simulink model "W01_S1"  (R2024b)
settings: Solver=ode4  StartTime=0  StopTime=T_final  FixedStep=h  RelTol=1e-3
undefined symbols (not defined in the file or in its folder): beta_c, mp, n0, rp, V_c, x0
settings Model: Creator=admin  LastModifiedBy=admin
settings DataIOCC: ReturnWorkspaceOutputs=off

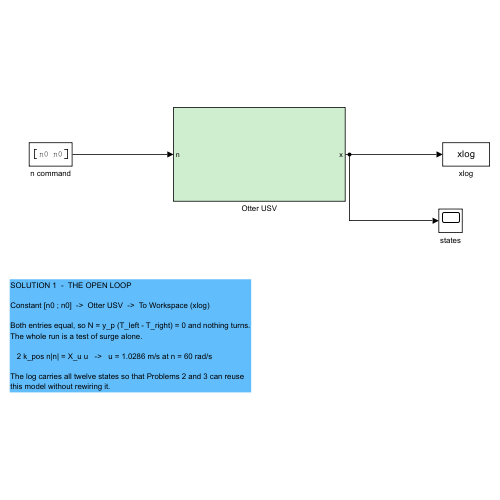
[thumbnail: Simulink's stored preview of the top-level diagram]
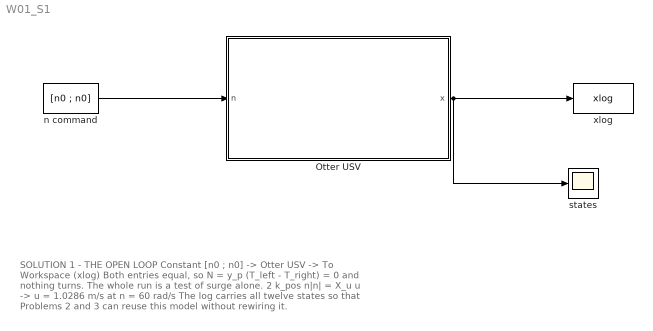
== system W01_S1 ==
  note: SOLUTION 1  -  THE OPEN LOOP
      |
      | Constant [n0 ; n0]  ->  Otter USV  ->  To Workspace (xlog)
      |
      | Both entries equal, so N = y_p (T_left - T_right) = 0 and nothing turns.
      | The whole run is a test of surge alone.
      |
      |    2 k_pos n|n| = X_u u   ->   u = 1.0286 m/s at n = 60 rad/s
      |
      | The log carries all twelve states so that Problems 2 and 3 can reuse
      | this model without rewiring it.
  Otter USV : Subsystem
  n command : Constant  Value=[n0 ; n0]
  states : Scope
  xlog : ToWorkspace  VariableName=xlog  SaveFormat=Structure With Time  SampleTime=-1
  wires:
  n command/1 -> Otter USV/1(n)
  Otter USV/1(x) -> xlog/1, states/1

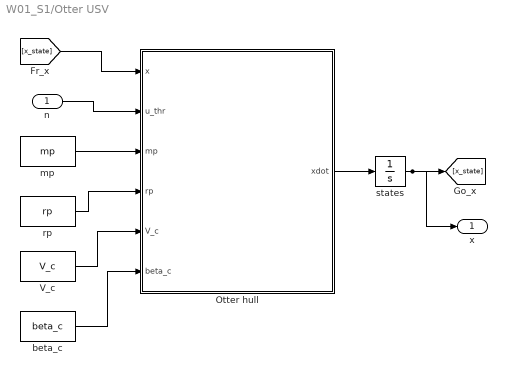
== system W01_S1/Otter USV ==
  n : Inport
  Otter hull : MATLAB Function  TreatAsAtomicUnit=on
  V_c : Constant  Value=V_c
  beta_c : Constant  Value=beta_c
  mp : Constant  Value=mp
  rp : Constant  Value=rp
  states : Integrator  InitialCondition=x0
  x : Outport
  wires:
  beta_c/1 -> Otter hull/6(beta_c)
  [x_state] -> Otter hull/1(x)
  rp/1 -> Otter hull/4(rp)
  mp/1 -> Otter hull/3(mp)
  n/1 -> Otter hull/2(u_thr)
  V_c/1 -> Otter hull/5(V_c)
  Otter hull/1(xdot) -> states/1
  states/1 -> [x_state], x/1

== matlab function W01_S1/Otter USV/Otter hull ==
  data: x input; xdot output double size=[12 1]; u_thr input; mp input; rp input; V_c input; beta_c input
function xdot = otter_hull(x, u_thr, mp, rp, V_c, beta_c)
% Fossen's otter.m, called unchanged from Tools/MSS/VESSELS.
%
%   x       12 states, fed back from the integrator
%   u_thr   propeller shaft speeds [rad/s]
%
% otter.m is not written for code generation, so the call is extrinsic and
% xdot has to be pre-sized for Simulink to know the output width.
coder.extrinsic('otter');

xdot = zeros(12,1);
xdot = otter(x, u_thr, mp, rp, V_c, beta_c);
end
